simulink model "model_validation_theta_CL_lab"  (R2023b)
settings: Solver=VariableStepAuto  StartTime=0.0  StopTime=100  RelTol=1e-3
values from neighbouring files (symbols this model uses):
  A = double(A)    [consistent.m]    (also in dyn_model_mark.m)
  B = double(B)    [consistent.m]    (also in dyn_model_mark.m)
  C = [1 0 0 0 ... (first row only)    [consistent.m]    (also in dyn_model_mark.m)
  D = [0 ... (first row only)    [consistent.m]    (also in dyn_model_mark.m)
  g0 = 9.81    [consistent.m]    (also in dyn_model_mark.m)
  Ip = (mp*Lp^2)/12    (= 3.3282e-05)    [consistent.m]    (also in dyn_model_mark.m = 8.3205e-06)
  Ir = (mr*Lr^2)/12    (= 5.71979166667e-05)    [consistent.m]    (also in dyn_model_mark.m = 1.42994791667e-05)
  K = place(A,B,P)    [consistent.m]    (also in dyn_model_mark.m)
  La = 1.16e-3    (= 0.00116)    [consistent.m]    (also in dyn_model_mark.m)
  Lp = 0.129    [consistent.m]    (also in dyn_model_mark.m = 0.0645)
  Lr = 0.085    [consistent.m]    (also in dyn_model_mark.m)
  mp = 0.024    [consistent.m]    (also in dyn_model_mark.m)
  mr = 0.095    [consistent.m]    (also in dyn_model_mark.m)
  phi_dot_init = 0    [consistent.m]
  phi_init = 0    [consistent.m]
  R_tilde = zeros(2,2)    [consistent.m]
  Ra = 8.4    [consistent.m]    (also in dyn_model_mark.m)
  theta_dot_init = 0    [consistent.m]
  theta_init = 0    [consistent.m]
undefined symbols (not defined in the file or in its folder): alfa, beta, Continuous, dist, Ir_tot, Ld, rot_pend, Time
libraries: simulink_extras x4, ctrlSharedLib x1
settings Model: Creator=Mark  LastModifiedBy=Mark

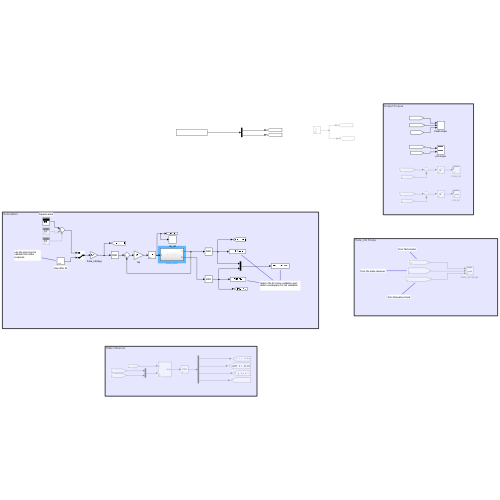
[thumbnail: Simulink's stored preview of the top-level diagram]
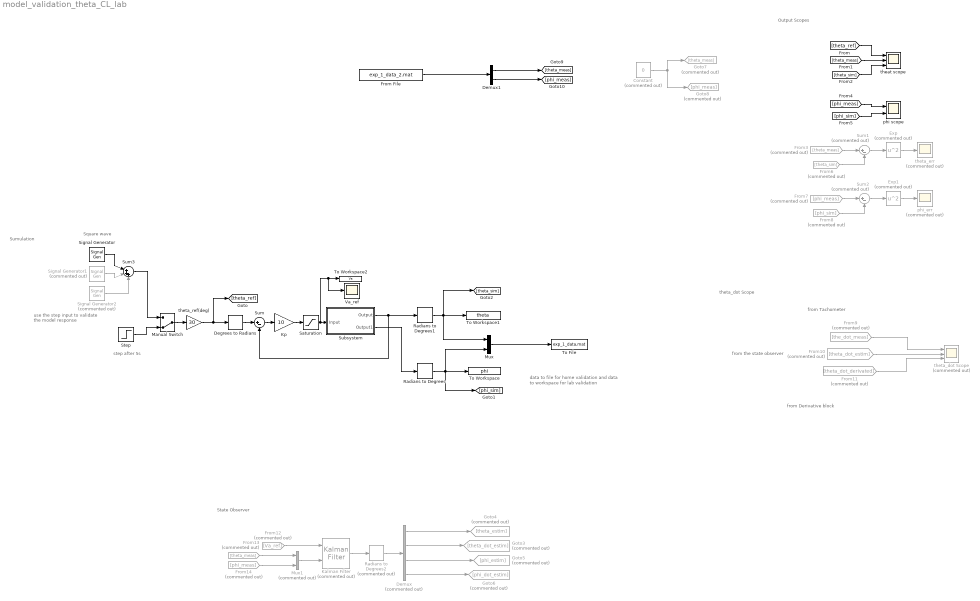
== system model_validation_theta_CL_lab ==
  note: State Observer
  note: Sumulation
  note: theta_dot Scope
  note: from Tachometer
  note: from Derivative block
  note: from the state observer
  note: Output Scopes
  note: use the step input to validate the model response
  note: data to file for home validation and data to workspace for lab validation
  note: step after 5s
  note: Square wave
  Constant : Constant  Commented=on  Value=0
  Degrees to Radians : simulink_extras/Transformations/Degrees to Radians
  Demux : Demux  Commented=on
  Demux1 : Demux  Outputs=2
  Exp : Math  Commented=on  Operator=square
  Exp1 : Math  Commented=on  Operator=square
  From File : FromFile  FileName=exp_1_data_2.mat  SampleTime=0
  From10 : From  Commented=on  GotoTag=theta_dot_estim
  From11 : From  Commented=on  GotoTag=theta_dot_derivated
  From12 : From  Commented=on  GotoTag=Va_ref
  From13 : From  Commented=on  GotoTag=theta_meas
  From14 : From  Commented=on  GotoTag=phi_meas
  From3 : From  Commented=on  GotoTag=theta_meas
  From6 : From  Commented=on  GotoTag=theta_sim
  From7 : From  Commented=on  GotoTag=phi_meas
  From8 : From  Commented=on  GotoTag=phi_sim
  From9 : From  Commented=on  GotoTag=the_dot_meas
  Goto3 : Goto  Commented=on  GotoTag=theta_dot_estim
  Goto4 : Goto  Commented=on  GotoTag=theta_estim
  Goto5 : Goto  Commented=on  GotoTag=phi_estim
  Goto6 : Goto  Commented=on  GotoTag=phi_dot_estim
  Goto7 : Goto  Commented=on  GotoTag=theta_meas
  Goto8 : Goto  Commented=on  GotoTag=phi_meas
  Kalman Filter : ctrlSharedLib/Kalman Filter  Commented=on  TimeDomain=Continuous-Time  UseCurrentEstimator=on  ModelSource=Individual A, B, C, D matrices  ModelSourceVariable=ss(0.95,1,1,0,1)  A=A  B=B  C=C  D=D  NumberOfStates=1  NumberOfInputs=1  NumberOfOutputs=1  InitialEstimateSource=Dialog  X0=[0 0 pi 0]  P0=10  UseK=off  UseGH=off  NumberOfProcessNoiseInputs=1  G=1  TimeInvariantG=on  H=0  TimeInvariantH=on  Q=Q_tilde  TimeInvariantQ=on  R=R_tilde  TimeInvariantR=on  N=0  TimeInvariantN=on  AddInputPort=on  AddEnablePort=off  OutputEstimatedY=off  OutputP=off  Ts=-1
  Kp : Gain  Gain=10
  Manual Switch : ManualSwitch  CurrentSetting=0
  Mux : Mux  Inputs=2
  Mux1 : Mux  Commented=on  Inputs=2
  Radians to Degrees : simulink_extras/Transformations/Radians to Degrees
  Radians to Degrees1 : simulink_extras/Transformations/Radians to Degrees
  Radians to Degrees2 : simulink_extras/Transformations/Radians to Degrees  Commented=on
  Saturation : Saturate  UpperLimit=10  LowerLimit=-10
  Signal Generator : SignalGenerator  WaveForm=square  Frequency=0.05
  Signal Generator1 : SignalGenerator  Commented=on  WaveForm=square  Frequency=0.5
  Signal Generator2 : SignalGenerator  Commented=on  WaveForm=square
  Step : Step  Time=5  SampleTime=0
  Subsystem : Subsystem
  Sum : Sum  Inputs=|+-
  Sum1 : Sum  Commented=on  Inputs=|+-
  Sum2 : Sum  Commented=on  Inputs=|+-
  Sum3 : Sum  Inputs=|+++
  To File : ToFile  Filename=exp_1_data.mat  MatrixName=angle
  To Workspace : ToWorkspace  VariableName=phi  SampleTime=-1
  To Workspace1 : ToWorkspace  VariableName=theta  SampleTime=-1
  To Workspace2 : ToWorkspace  VariableName=Va  SampleTime=-1
  Va_ref : Scope
  phi scope : Scope  NumInputPorts=2
  phi_err : Scope  Commented=on
  theat scope : Scope  NumInputPorts=3
  theta_dot Scope : Scope  Commented=on  NumInputPorts=3
  theta_err : Scope  Commented=on
  theta_ref(deg) : Gain  Gain=30
  wires:
  Mux/1 -> To File/1
  Kp/1 -> Saturation/1
  Saturation/1 -> Va_ref/1, To Workspace2/1, Subsystem/1(Input)
  Step/1 -> Manual Switch/2
  theta_ref(deg)/1 -> [theta_ref], Degrees to Radians/1
  Radians to Degrees1/1 -> [theta_sim], To Workspace1/1, Mux/1
  Degrees to Radians/1 -> Sum/1
  Subsystem/2(Output1) -> Radians to Degrees/1
  Radians to Degrees/1 -> Mux/2, To Workspace/1, [phi_sim]
  Subsystem/1(Output) -> Radians to Degrees1/1, Sum/2
  Sum/1 -> Kp/1
  Manual Switch/1 -> theta_ref(deg)/1
  [theta_meas] -> theat scope/2
  [theta_sim] -> theat scope/3
  [theta_ref] -> theat scope/1
  [phi_meas] -> phi scope/1
  [phi_sim] -> phi scope/2
  Exp/1 -> theta_err/1
  Sum1/1 -> Exp/1
  From3/1 -> Sum1/1
  From6/1 -> Sum1/2
  From8/1 -> Sum2/2
  Exp1/1 -> phi_err/1
  Sum2/1 -> Exp1/1
  From7/1 -> Sum2/1
  From9/1 -> theta_dot Scope/1
  From10/1 -> theta_dot Scope/2
  From11/1 -> theta_dot Scope/3
  Radians to Degrees2/1 -> Demux/1
  Kalman Filter/1 -> Radians to Degrees2/1
  Mux1/1 -> Kalman Filter/2
  From12/1 -> Kalman Filter/1
  From13/1 -> Mux1/1
  From14/1 -> Mux1/2
  Demux/2 -> Goto3/1
  Demux/1 -> Goto4/1
  Demux/3 -> Goto5/1
  Demux/4 -> Goto6/1
  Constant/1 -> Goto8/1, Goto7/1
  From File/1 -> Demux1/1
  Demux1/1 -> [theta_meas]
  Demux1/2 -> [phi_meas]
  Sum3/1 -> Manual Switch/1
  Signal Generator/1 -> Sum3/1
  Signal Generator1/1 -> Sum3/2
  Signal Generator2/1 -> Sum3/3

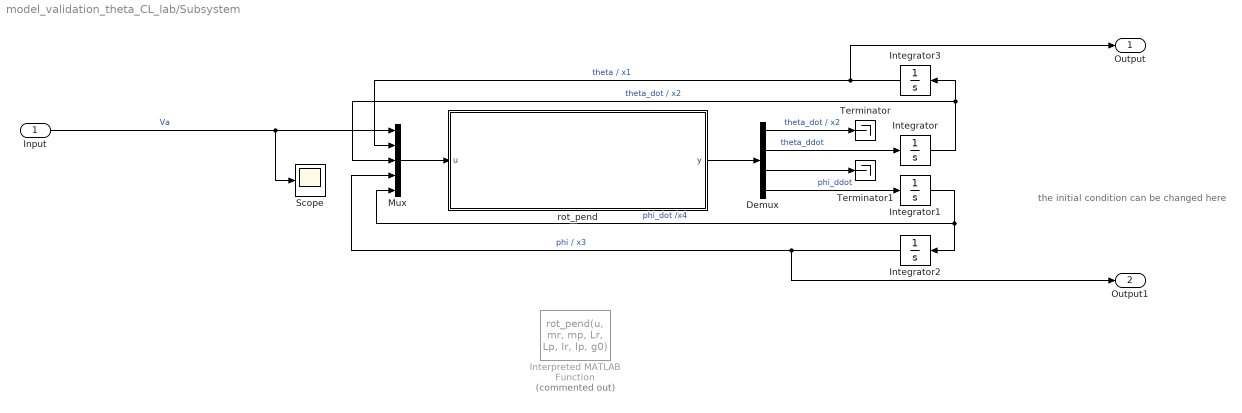
== system model_validation_theta_CL_lab/Subsystem ==
  note: the initial condition can be changed here
  Input : Inport
  Demux : Demux
  Integrator : Integrator  InitialCondition=theta_dot_init
  Integrator1 : Integrator  InitialCondition=phi_dot_init
  Integrator2 : Integrator  InitialCondition=phi_init
  Integrator3 : Integrator  InitialCondition=theta_init
  Interpreted MATLAB Function : MATLABFcn  Commented=on  MATLABFcn=rot_pend(u, mr, mp, Lr, Lp, Ir, Ip, g0)  OutputDimensions=4  OutputSignalType=real
  Mux : Mux  Inputs=5
  Scope : Scope
  Terminator : Terminator
  Terminator1 : Terminator
  rot_pend : Subsystem
  Output : Outport
  Output1 : Outport  Port=2
  wires:
  Input/1 -> Scope/1, Mux/1  "Va"
  Integrator2/1 -> Output1/1, Mux/4  "phi / x3"
  Integrator/1 -> Integrator3/1, Mux/3  "theta_dot / x2"
  Mux/1 -> rot_pend/1(u)
  rot_pend/1(y) -> Demux/1
  Integrator1/1 -> Mux/5, Integrator2/1  "phi_dot /x4"
  Integrator3/1 -> Mux/2, Output/1  "theta / x1"
  Demux/4 -> Integrator1/1  "phi_ddot"
  Demux/2 -> Integrator/1  "theta_ddot"
  Demux/1 -> Terminator/1  "theta_dot / x2"
  Demux/3 -> Terminator1/1

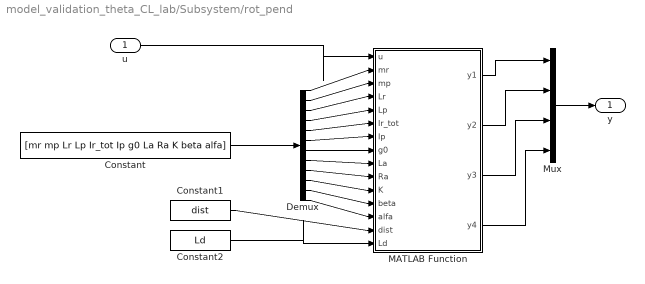
== system model_validation_theta_CL_lab/Subsystem/rot_pend ==
  u : Inport
  Constant : Constant  Value=[mr mp Lr Lp Ir_tot Ip g0 La Ra K beta alfa]  VectorParams1D=off
  Constant1 : Constant  Value=dist
  Constant2 : Constant  Value=Ld
  Demux : Demux  Outputs=12
  MATLAB Function : MATLAB Function  TreatAsAtomicUnit=on
  Mux : Mux
  y : Outport
  wires:
  Demux/3 -> MATLAB Function/4(Lr)
  Demux/5 -> MATLAB Function/6(Ir_tot)
  Demux/4 -> MATLAB Function/5(Lp)
  Demux/7 -> MATLAB Function/8(g0)
  Demux/2 -> MATLAB Function/3(mp)
  Demux/6 -> MATLAB Function/7(Ip)
  Demux/1 -> MATLAB Function/2(mr)
  u/1 -> MATLAB Function/1(u)
  Constant/1 -> Demux/1
  MATLAB Function/1(y1) -> Mux/1
  MATLAB Function/2(y2) -> Mux/2
  MATLAB Function/3(y3) -> Mux/3
  MATLAB Function/4(y4) -> Mux/4
  Mux/1 -> y/1
  Demux/8 -> MATLAB Function/9(La)
  Demux/9 -> MATLAB Function/10(Ra)
  Demux/10 -> MATLAB Function/11(K)
  Demux/11 -> MATLAB Function/12(beta)
  Demux/12 -> MATLAB Function/13(alfa)
  Constant1/1 -> MATLAB Function/14(dist)
  Constant2/1 -> MATLAB Function/15(Ld)

== matlab function model_validation_theta_CL_lab/Subsystem/rot_pend/MATLAB Function ==
  data: u input; y1 output; mr input; mp input; Lr input; Lp input; Ir_tot input; Ip input; g0 input; La input; Ra input; y2 output; y3 output; y4 output; K input; beta input; alfa input; dist input; Ld input
function [y1,y2,y3,y4] = rot_pend(u, mr, mp, Lr, Lp, Ir_tot, Ip, g0,La, Ra, K, beta,alfa, dist, Ld)
%UNTITLED Summary of this function goes here
%   Detailed explanation goes here
% u(1) = Va
x1 = u(2) ; % theta
x2 = u(3) ; % theta_dot
x3 = u(4) ; % phi
x4 = u(5) ; % phi_dot

H = [(mp*(Lr^2+((Lp/2)^2*(sin(x3))^2)))+Ir_tot            -mp*Lr*Lp*cos(x3)/2;
                     -mp*Lr*Lp*cos(x3)/2                              (mp*(Lp/2)^2)+Ip] ;

Q = [mp*(Lp/2)^2*sin(x3)*cos(x3)*x4+beta                      (mp*(Lp/2)^2*sin(x3)*cos(x3)*x2)-(mp*Lr*(Lp/2)*sin(x3)*x4);
     -mp*(Lp/2)^2*sin(x3)*cos(x3)*x2                                                   alfa                                   ] ;

g = [           0     ;
     mp*g0*(Lp/2)*sin(x3)] ;
%(K*u(1)/Ra)-(K^2*x2/Ra)
tau = [(K/Ra)*(u(1)-(K*x2)) ;
       0 ] ;

if (x1>=0.1745 | x1<=-0.1745)       % 0.08727rad = 5deg
     kt = 0.03 ;                    % 0.1745rad = 10deg
     kc = 10e-3 ;
else                               % 0.349rad = 20deg
    kt = 0 ;
    kc = 3.5e-3 ;
end

Tr_theta = ((kt*x1)+(kc*x2))*Ld ;

q_ddot = H\[tau - Q*[x2 x4]' - g - 1*[Tr_theta 0]' ] ;



y1 = x2 ;
y2 = q_ddot(1) ;
y3 = x4 ;
y4 = q_ddot(2) ;


%Ir+mr*(Lr/2)^2)
